simulink model "verify_PMV_PPD_mdl"  (R2016b)
settings: Solver=VariableStepDiscrete  StartTime=0  StopTime=1  MaxStep=1  RelTol=1e-3  EnableMultiTasking=on
libraries: carnot x1
settings Model: Creator=drhf  LastModifiedBy=drhf
settings DataIOCC: SaveFormat=Array  SignalLoggingSaveFormat=ModelDataLogs
settings OptimizationCC: ExpressionDepthLimit=2147483647  LifeSpan=inf
settings DebuggingCC: UnderspecifiedInitializationDetection=Classic  MergeDetectMultiDrivingBlocksExec=none  SolverPrmCheckMsg=warning  FcnCallInpInsideContextMsg=warning  StateNameClashWarn=warning  SFUnexpectedBacktrackingDiag=warning  SFNoUnconditionalDefaultTransitionDiag=warning  SFExecutionAtInitializationDiag=none
settings HardwareCC: ProdBitPerPointer=32  ProdBitPerSizeT=32  ProdBitPerPtrDiffT=32  ProdLargestAtomicFloat=None  ProdIntDivRoundTo=Undefined  ProdEndianess=Unspecified  ProdWordSize=32  ProdHWDeviceType=32-bit Generic
settings ModelReferenceCC: PropagateSignalLabelsOutOfModel=off
settings GRTTargetCC: TargetLangStandard=C89/C90 (ANSI)  GeneratePreprocessorConditionals=Disable all  CombineOutputUpdateFcns=off  GRTInterface=on
settings ConfigComp: CovMetricSettings=dw  CovHtmlReporting=on  CovSaveCumulativeToWorkspaceVar=on  CovSaveSingleToWorkspaceVar=on  CovExternalEMLEnable=off

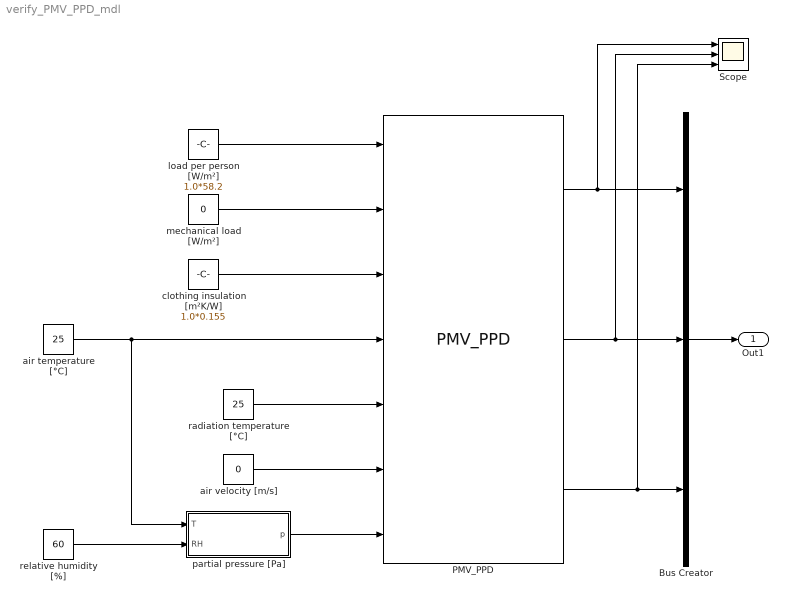
== system verify_PMV_PPD_mdl ==
  Bus Creator : BusCreator  Inputs=3
  PMV_PPD : carnot/Outputs/PMV_PPD  DEBUGLEVEL=WARNINGLEVEL  MAXTOTALWARNINGS=inf  MAXCONSECUTIVEWARNINGS=inf  WRITETOFILE=0  FILENAME='messages.txt'
  Scope : Scope  NumInputPorts=3
  air temperature [°C] : Constant  Value=25
  air velocity [m/s] : Constant  Value=0
  clothing insulation [m²K/W] : Constant  Value=1.0*0.155
  load per person [W/m²] : Constant  Value=1.0*58.2
  mechanical load [W/m²] : Constant  Value=0
  partial pressure [Pa] : Subsystem
  radiation temperature [°C] : Constant  Value=25
  relative humidity [%] : Constant  Value=60
  Out1 : Outport
  wires:
  Bus Creator/1 -> Out1/1
  PMV_PPD/2 -> Scope/2, Bus Creator/2
  PMV_PPD/1 -> Scope/1, Bus Creator/1
  PMV_PPD/3 -> Scope/3, Bus Creator/3
  mechanical load [W/m²]/1 -> PMV_PPD/2
  load per person [W/m²]/1 -> PMV_PPD/1
  clothing insulation [m²K/W]/1 -> PMV_PPD/3
  air temperature [°C]/1 -> partial pressure [Pa]/1(T), PMV_PPD/4
  relative humidity [%]/1 -> partial pressure [Pa]/2(RH)
  partial pressure [Pa]/1(p) -> PMV_PPD/7
  air velocity [m/s]/1 -> PMV_PPD/6
  radiation temperature [°C]/1 -> PMV_PPD/5

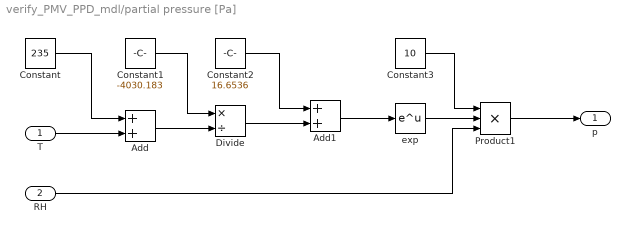
== system verify_PMV_PPD_mdl/partial pressure [Pa] ==
  T : Inport
  RH : Inport  Port=2
  Add : Sum
  Add1 : Sum
  Constant : Constant  Value=235
  Constant1 : Constant  Value=-4030.183
  Constant2 : Constant  Value=16.6536
  Constant3 : Constant  Value=10
  Divide : Product  Inputs=*/
  Product1 : Product  Inputs=3
  exp : Math  SaturateOnIntegerOverflow=on
  p : Outport
  wires:
  Constant/1 -> Add/1
  T/1 -> Add/2
  Add/1 -> Divide/2
  Constant1/1 -> Divide/1
  Divide/1 -> Add1/2
  Constant2/1 -> Add1/1
  Add1/1 -> exp/1
  exp/1 -> Product1/2
  RH/1 -> Product1/3
  Constant3/1 -> Product1/1
  Product1/1 -> p/1
